simulink model "model8krataA"  (Simulink 6.6)
settings: Solver=ode45  StartTime=0.0  StopTime=250.0  MaxStep=0.1  MinStep=0.01  RelTol=1e-6
values from neighbouring files (symbols this model uses):
  a1 = w1/w0    (= 84)    [dane8Krata.m]
  a2 = w2/w0    (= 273)    [dane8Krata.m]
  a3 = 1/w0    (= 180)    [dane8Krata.m]
  b0 = d12*d23 / (C1*w0)    (= 3)    [dane8Krata.m]
  kg = 42.1    [dane8Krata.m]
settings Model: Creator=Administrator  LastModifiedBy=Damian
settings DataIOCC: LimitDataPoints=off
settings GRTTargetCC: TargetFcnLib=ansi_tfl_table_tmw.mat

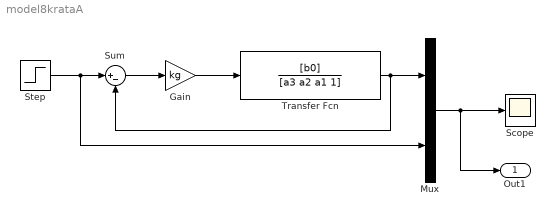
== system model8krataA ==
  Gain : Gain  Gain=kg
  Mux : Mux  Inputs=2
  Scope : Scope
  Step : Step  Time=0  SampleTime=0
  Sum : Sum  Inputs=|+-
  Transfer Fcn : TransferFcn  Numerator=[b0]  Denominator=[a3 a2 a1 1]
  Out1 : Outport
  wires:
  Mux/1 -> Scope/1, Out1/1
  Transfer Fcn/1 -> Sum/2, Mux/1
  Step/1 -> Sum/1, Mux/2
  Sum/1 -> Gain/1
  Gain/1 -> Transfer Fcn/1
